simulink model "fixedWingPath"  (R2023b)
settings: Solver=FixedStepAuto  StartTime=0.0  StopTime=70  FixedStep=0.01  RelTol=1e-3
model workspace: external: MATLAB File variable.m (data not in the file)
undefined symbols (not defined in the file or in its folder): DiscIntNeverNeededParam, LOGPOSX, POSY, Tgps, Tneuro, VarImu, VarNeuro
libraries: simulink x2, embmathops x2, uavalgslib x2, robotcorelib x1, uavutilslib x1
(part 1 of 2)
settings Model: DataDictionary=fixedWingPathFollowingData.sldd  EnableAccessToBaseWorkspace=off  PacingRate=10  Creator=The MathWorks, Inc.  LastModifiedBy=Utilisateur
settings SolverCC: AlgebraicLoopSolver=TrustRegion  DecoupledContinuousIntegration=on
settings DataIOCC: ReturnWorkspaceOutputs=off
settings OptimizationCC: ReuseModelBlockBuffer=off
settings DebuggingCC: UnconnectedInputMsg=warning  UnconnectedOutputMsg=warning  UnconnectedLineMsg=warning  ArithmeticOperatorsInVariantConditions=warning
settings ModelReferenceCC: EnableRefExpFcnMdlSchedulingChecks=on
settings SFSimCC: SimUseLocalCustomCode=off  CustomCodeUndefinedFunction=UseInterfaceOnly
settings RTWCC: RTWUseLocalCustomCode=off  DLArmComputeVersion=19.05

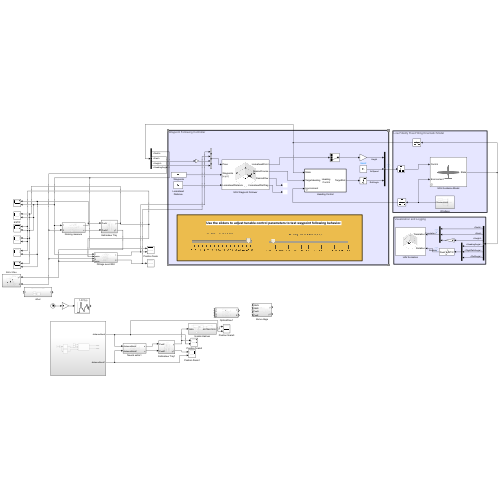
[thumbnail: Simulink's stored preview of the top-level diagram]
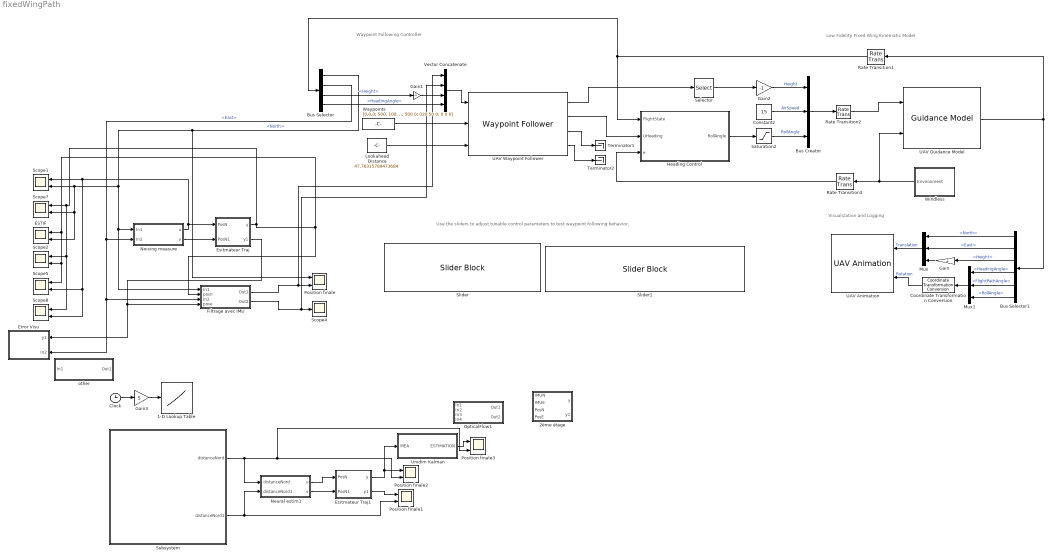
== system fixedWingPath ==
  note: Use the sliders to adjust tunable control parameters to test waypoint following behavior.
  note: Visualization and Logging
  note: Low Fidelity Fixed Wing Kinematic Model
  note: Waypoint Following Controller
  1-D Lookup Table : Lookup_n-D  NumberOfTableDimensions=1  BreakpointsForDimension1=1:337  Table=LOGPOSX  InternalRulePriority=Speed  RndMeth=Simplest
  2ème étage : Subsystem
  Bus Creator : BusCreator  Inputs=3  OutDataTypeStr=Bus: FixedWingControlBus  NonVirtualBus=on
  Bus Selector : BusSelector  OutputSignals=North,East,Height,HeadingAngle
  Bus Selector1 : BusSelector  OutputSignals=North,East,Height,HeadingAngle,FlightPathAngle,RollAngle
  Clock : Clock
  Constant2 : Constant  Value=15
  Coordinate Transformation Conversion : robotcorelib/Coordinate Transformation Conversion  InputRepresentation=Euler Angles  InputEulerSequence=ZYX  ShowTrVecInputPort=on  OutputRepresentation=Quaternion  OutputEulerSequence=ZYX  ShowTrVecOutputPort=on  SimulateUsing=Code generation
  ESTIF : Scope  NumInputPorts=2
  Error Visu : Subsystem
  Esitmateur Traj : Subsystem
  Esitmateur Traj1 : Subsystem
  Filtrage avec IMU : Subsystem
  Gain : Gain  Gain=-1
  Gain1 : Gain  Gain=-1
  Gain2 : Gain  Gain=-1
  Gain3 : Gain  Gain=5
  Heading Control : MATLAB Function  TreatAsAtomicUnit=on  mask(Fixed Wing Heading Controller){PHeadingAngle=0.5997978032950574}
      mask prompts: PHeadingAngle "Heading Control Gain"
      mask help: P controller that regulates fixed wing UAV heading direction through controlling its roll angle. This controller requires that the plane is flying under coordinated flight condition.
  Lookahead Distance : Constant  Value=47.76315789473684
  Mux : Mux  Inputs=3
  Mux1 : Mux  Inputs=3
  Neural estim1 : Subsystem
  Noising measure : Subsystem
  OpticalFlow1 : Subsystem
  Position finale{,1..3} (4 alike) : Scope  NumInputPorts=2
  Rate Transition1 : RateTransition  OutPortSampleTime=0.01
  Rate Transition2 : RateTransition  OutPortSampleTime=0.1
  Rate Transition3 : RateTransition  OutPortSampleTime=0.01
  Saturation2 : Saturate  UpperLimit=20/180*pi  LowerLimit=-20/180*pi
  Scope{1..2,5,7..8} (5 alike) : Scope  NumInputPorts=2
  Scope4 : Scope
  Selector : Selector  InputPortWidth=3  IndexOptions=Index vector (dialog)  Indices=[3]  OutputSizes=1
  Slider : SliderBlock  ScaleMin=5  ScaleMax=50
  Slider1 : SliderBlock  ScaleMin=0.39000000000000001  ScaleMax=3.8999999999999999
  Subsystem : Subsystem
  Terminator1 : Terminator
  Terminator2 : Terminator
  UAV Animation : uavutilslib/UAV Animation  UAVType=FixedWing  UAVSize=50  InertialZDirection=Down  SampleTime=0.1
  UAV Guidance Model : uavalgslib/Guidance Model  ModelType=FixedWingGuidance  SpecifiedDataType=double  SimulateUsing=Code generation  InitialWorldPositionMultirotor=[0; 0; 0]  InitialWorldVelocityMultirotor=[0; 0; 0]  InitialEulerZYXMultirotor=[0; 0; 0]  InitialBodyAngularRateRPYMultirotor=[0; 0; 0]  InitialThrustMultirotor=0  InitialNorthFixedWing=0  InitialEastFixedWing=0  InitialHeightFixedWing=0  InitialAirSpeedFixedWing=15  InitialHeadingAngleFixedWing=0  InitialFlightPathAngleFixedWing=0  InitialRollAngleFixedWing=0  InitialRollAngleRateFixedWing=0  PDRollMultirotor=[3402.97,116.67]  PDPitchMultirotor=[3402.97, 116.67]  PYawRateMultirotor=1950  PThrustMultirotor=3900  MassMultirotor=0.1  PHeightFixedWing=3.9  PHeadingAngleFixedWing=3.9  PFlightPathAngleFixedWing=39  PDRollFixedWing=[5.9414, 3.9]  PAirSpeedFixedWing=1  FlightPathAngleLimitsFixedWing=[-pi/6, pi/6]  StateBusName='FixedWingStateBus'  ControlBusName='FixedWingControlBus'  EnvironmentBusName='FixedWingEnvironmentBus'  DataType=double
  UAV Waypoint Follower : uavalgslib/Waypoint Follower  UAVType=fixed-wing  StartFrom=first  TransitionRadiusSource=internal  TransitionRadius=10  MinLookaheadDistance=0.1  YawInput=off  ShowCrossTrackErrorOutput=off  ShowStatusOutput=off  SimulateUsing=Code generation
  Unidim Kalman : Subsystem
  Vector Concatenate : Concatenate  NumInputs=4
  Waypoints : Constant  Value=[0,0,0; 500, 100, 3; 500, 500, 0; 020 500 0; 020 50 0; 0 0 0]  VectorParams1D=off
  Windless : Subsystem  VariantControl=NoWind
  other : Subsystem
  wires:
  Constant2/1 -> Bus Creator/2  "AirSpeed"
  Gain2/1 -> Bus Creator/1  "Height"
  Bus Creator/1 -> Rate Transition2/1
  Bus Selector/1 -> Position finale/1, ESTIF/2, Scope7/2, Scope1/2, Filtrage avec IMU/1(In1), Noising measure/1(In1)  "<North>"
  Bus Selector/2 -> Error Visu/2(In2), Filtrage avec IMU/3(In2), Noising measure/2(In2)  "<East>"
  Saturation2/1 -> Bus Creator/3  "RollAngle"
  Rate Transition1/1 -> Heading Control/1(FlightState), Bus Selector/1
  Rate Transition2/1 -> UAV Guidance Model/1
  UAV Waypoint Follower/2 -> Heading Control/2(UHeading)
  UAV Waypoint Follower/1 -> Selector/1
  Waypoints/1 -> UAV Waypoint Follower/2
  Vector Concatenate/1 -> UAV Waypoint Follower/1
  UAV Waypoint Follower/3 -> Terminator1/1
  Lookahead Distance/1 -> UAV Waypoint Follower/3
  Heading Control/1(RollAngle) -> Saturation2/1
  Gain/1 -> Mux/3
  Bus Selector1/6 -> Mux1/3  "<RollAngle>"
  Bus Selector1/5 -> Mux1/2  "<FlightPathAngle>"
  Mux1/1 -> Coordinate Transformation Conversion/1
  Coordinate Transformation Conversion/1 -> UAV Animation/2  "Rotation"
  UAV Guidance Model/1 -> Bus Selector1/1, Rate Transition1/1
  Mux/1 -> UAV Animation/1  "Translation"
  Windless/1(Environment) -> UAV Guidance Model/2, Rate Transition3/1
  Bus Selector/4 -> Vector Concatenate/4  "<HeadingAngle>"
  Bus Selector/3 -> Gain1/1  "<Height>"
  Gain1/1 -> Vector Concatenate/3
  Selector/1 -> Gain2/1
  Rate Transition3/1 -> Heading Control/3(e)
  Bus Selector1/1 -> Mux/1  "<North>"
  Bus Selector1/2 -> Mux/2  "<East>"
  Bus Selector1/4 -> Mux1/1  "<HeadingAngle>"
  Bus Selector1/3 -> Gain/1  "<Height>"
  UAV Waypoint Follower/4 -> Terminator2/1
  Filtrage avec IMU/1(Out1) -> Vector Concatenate/1, Position finale/2
  Filtrage avec IMU/2(Out2) -> Vector Concatenate/2, Scope4/1
  Noising measure/1(u) -> Scope8/2, Scope5/2, Scope1/1, Esitmateur Traj/1(PosN)
  Noising measure/2(v) -> Esitmateur Traj/2(PosN1)
  Esitmateur Traj/1(y) -> Scope8/1, Scope2/1, Scope7/1, Scope5/1, Scope2/2, ESTIF/1, Filtrage avec IMU/2(posn)
  Esitmateur Traj/2(y1) -> Filtrage avec IMU/4(pose), Error Visu/1(y1)
  Neural estim1/1(u) -> Esitmateur Traj1/1(PosN)
  Clock/1 -> Gain3/1
  Gain3/1 -> 1-D Lookup Table/1
  Esitmateur Traj1/1(y) -> Unidim Kalman/1(MEA), Position finale2/1
  Esitmateur Traj1/2(y1) -> Position finale1/1
  Neural estim1/2(v) -> Esitmateur Traj1/2(PosN1)
  Subsystem/1(distanceNord) -> Neural estim1/1(distanceNord), Position finale3/2, Position finale2/2
  Subsystem/2(distanceNord1) -> Position finale1/2, Neural estim1/2(distanceNord1)
  Unidim Kalman/1(ESTIMATION) -> Position finale3/1

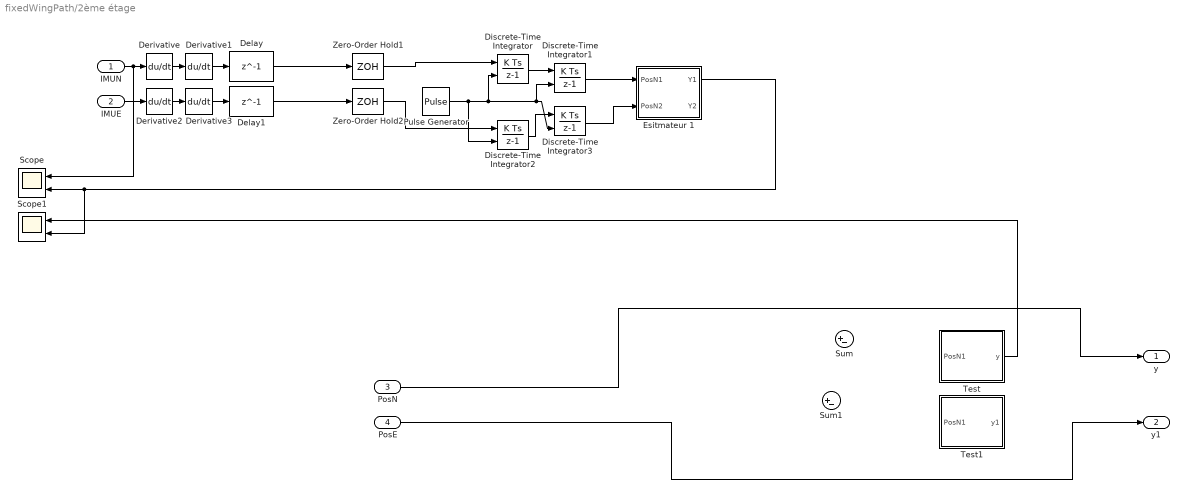
== system fixedWingPath/2ème étage ==
  IMUN : Inport
  IMUE : Inport  Port=2
  PosN : Inport  Port=3
  PosE : Inport  Port=4
  Delay : Delay  DelayLength=1  InitialCondition=0  SampleTime=0.05
  Delay1 : Delay  DelayLength=1  InitialCondition=0  SampleTime=0.05
  Derivative{,1..3} (4 alike) : Derivative
  Discrete-Time Integrator{,1..3} (4 alike) : DiscreteIntegrator  ExternalReset=rising  SampleTime=0.1  ICPrevOutput=DiscIntNeverNeededParam  ICPrevScaledInput=DiscIntNeverNeededParam
  Esitmateur 1 : Subsystem
  Pulse Generator : DiscretePulseGenerator  PulseType=Time based  Period=Tneuro  PulseWidth=50
  Scope : Scope  NumInputPorts=2
  Scope1 : Scope  NumInputPorts=2
  Sum : Sum  Inputs=|+-
  Sum1 : Sum  Inputs=|+-
  Test : Subsystem
  Test1 : Subsystem
  Zero-Order Hold1 : ZeroOrderHold  SampleTime=Tgps
  Zero-Order Hold2 : ZeroOrderHold  SampleTime=Tgps
  y : Outport
  y1 : Outport  Port=2
  wires:
  Zero-Order Hold1/1 -> Discrete-Time Integrator/1
  Derivative1/1 -> Delay/1
  Derivative/1 -> Derivative1/1
  IMUN/1 -> Scope/1, Derivative/1
  Derivative3/1 -> Delay1/1
  Zero-Order Hold2/1 -> Discrete-Time Integrator2/1
  IMUE/1 -> Derivative2/1
  Derivative2/1 -> Derivative3/1
  Pulse Generator/1 -> Discrete-Time Integrator2/2, Discrete-Time Integrator3/2, Discrete-Time Integrator1/2, Discrete-Time Integrator/2
  Discrete-Time Integrator/1 -> Discrete-Time Integrator1/1
  Discrete-Time Integrator2/1 -> Discrete-Time Integrator3/1
  Discrete-Time Integrator1/1 -> Esitmateur 1/1(PosN1)
  Discrete-Time Integrator3/1 -> Esitmateur 1/2(PosN2)
  Esitmateur 1/1(Y1) -> Scope1/2, Scope/2
  Delay/1 -> Zero-Order Hold1/1
  Delay1/1 -> Zero-Order Hold2/1
  Test/1(y) -> Scope1/1
  PosN/1 -> y/1
  PosE/1 -> y1/1

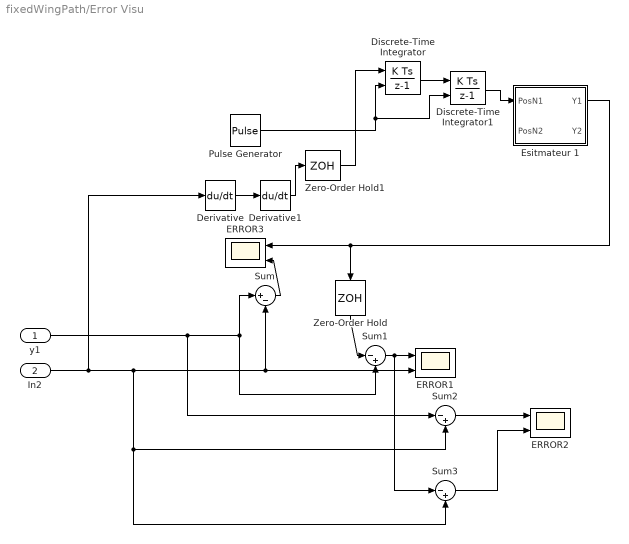
== system fixedWingPath/Error Visu ==
  y1 : Inport
  In2 : Inport  Port=2
  Derivative : Derivative
  Derivative1 : Derivative
  Discrete-Time Integrator : DiscreteIntegrator  ExternalReset=rising  SampleTime=0.1  ICPrevOutput=DiscIntNeverNeededParam  ICPrevScaledInput=DiscIntNeverNeededParam
  Discrete-Time Integrator1 : DiscreteIntegrator  ExternalReset=rising  SampleTime=0.1  ICPrevOutput=DiscIntNeverNeededParam  ICPrevScaledInput=DiscIntNeverNeededParam
  ERROR1 : Scope  NumInputPorts=2
  ERROR2 : Scope  NumInputPorts=2
  ERROR3 : Scope  NumInputPorts=2
  Esitmateur 1 : Subsystem
  Pulse Generator : DiscretePulseGenerator  PulseType=Time based  Period=Tneuro  PulseWidth=50
  Sum : Sum  Inputs=|+-
  Sum1 : Sum  Inputs=|-+
  Sum2 : Sum  Inputs=|-+
  Sum3 : Sum  Inputs=|-+
  Zero-Order Hold : ZeroOrderHold  SampleTime=Tgps
  Zero-Order Hold1 : ZeroOrderHold  SampleTime=Tgps
  wires:
  Sum/1 -> ERROR3/2
  y1/1 -> Sum/1, Sum1/2, Sum2/1
  In2/1 -> Sum2/2, Sum3/2, ERROR1/2, Sum/2, Derivative/1
  Derivative1/1 -> Zero-Order Hold1/1
  Sum1/1 -> Sum3/1, ERROR1/1
  Zero-Order Hold/1 -> Sum1/1
  Derivative/1 -> Derivative1/1
  Zero-Order Hold1/1 -> Discrete-Time Integrator/1
  Sum2/1 -> ERROR2/1
  Sum3/1 -> ERROR2/2
  Discrete-Time Integrator/1 -> Discrete-Time Integrator1/1
  Pulse Generator/1 -> Discrete-Time Integrator/2, Discrete-Time Integrator1/2
  Discrete-Time Integrator1/1 -> Esitmateur 1/1(PosN1)
  Esitmateur 1/1(Y1) -> Zero-Order Hold/1, ERROR3/1

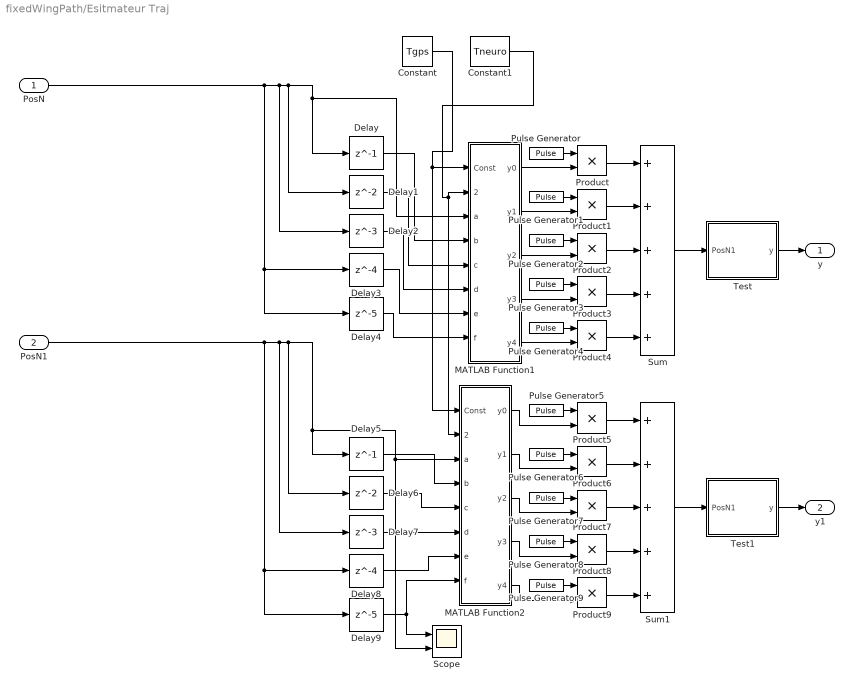
== system fixedWingPath/Esitmateur Traj ==
  PosN : Inport
  PosN1 : Inport  Port=2
  Constant : Constant  Value=Tgps
  Constant1 : Constant  Value=Tneuro
  Delay : Delay  DelayLength=1  SampleTime=Tneuro
  Delay1 : Delay  SampleTime=Tneuro
  Delay2 : Delay  DelayLength=3  SampleTime=Tneuro
  Delay3 : Delay  DelayLength=4  SampleTime=Tneuro
  Delay4 : Delay  DelayLength=5  SampleTime=Tneuro
  Delay5 : Delay  DelayLength=1  SampleTime=Tneuro
  Delay6 : Delay  SampleTime=Tneuro
  Delay7 : Delay  DelayLength=3  SampleTime=Tneuro
  Delay8 : Delay  DelayLength=4  SampleTime=Tneuro
  Delay9 : Delay  DelayLength=5  SampleTime=Tneuro
  MATLAB Function1 : MATLAB Function  TreatAsAtomicUnit=on
  MATLAB Function2 : MATLAB Function  TreatAsAtomicUnit=on
  Product{,1..9} (10 alike) : Product
  Pulse Generator : DiscretePulseGenerator  PulseType=Time based  Period=Tneuro  PulseWidth=20
  Pulse Generator1 : DiscretePulseGenerator  PulseType=Time based  Period=Tneuro  PulseWidth=20  PhaseDelay=0.2*Tneuro
  Pulse Generator2 : DiscretePulseGenerator  PulseType=Time based  Period=Tneuro  PulseWidth=20  PhaseDelay=0.4*Tneuro
  Pulse Generator3 : DiscretePulseGenerator  PulseType=Time based  Period=Tneuro  PulseWidth=20  PhaseDelay=0.6*Tneuro
  Pulse Generator4 : DiscretePulseGenerator  PulseType=Time based  Period=Tneuro  PulseWidth=20  PhaseDelay=0.8*Tneuro
  Pulse Generator5 : DiscretePulseGenerator  PulseType=Time based  Period=Tneuro  PulseWidth=20
  Pulse Generator6 : DiscretePulseGenerator  PulseType=Time based  Period=Tneuro  PulseWidth=20  PhaseDelay=0.2*Tneuro
  Pulse Generator7 : DiscretePulseGenerator  PulseType=Time based  Period=Tneuro  PulseWidth=20  PhaseDelay=0.4*Tneuro
  Pulse Generator8 : DiscretePulseGenerator  PulseType=Time based  Period=Tneuro  PulseWidth=20  PhaseDelay=0.6*Tneuro
  Pulse Generator9 : DiscretePulseGenerator  PulseType=Time based  Period=Tneuro  PulseWidth=20  PhaseDelay=0.8*Tneuro
  Scope : Scope  NumInputPorts=2
  Sum : Sum  Inputs=+++++
  Sum1 : Sum  Inputs=+++++
  Test : Subsystem
  Test1 : Subsystem
  y : Outport
  y1 : Outport  Port=2
  wires:
  Delay/1 -> MATLAB Function1/4(b)
  Delay1/1 -> MATLAB Function1/5(c)
  Delay2/1 -> MATLAB Function1/6(d)
  Delay3/1 -> MATLAB Function1/7(e)
  Delay4/1 -> MATLAB Function1/8(f)
  Product/1 -> Sum/1
  Product1/1 -> Sum/2
  Product2/1 -> Sum/3
  Product3/1 -> Sum/4
  Product4/1 -> Sum/5
  Pulse Generator/1 -> Product/1
  Pulse Generator1/1 -> Product1/1
  Pulse Generator2/1 -> Product2/1
  Pulse Generator3/1 -> Product3/1
  Pulse Generator4/1 -> Product4/1
  MATLAB Function1/1(y0) -> Product/2
  MATLAB Function1/2(y1) -> Product1/2
  MATLAB Function1/3(y2) -> Product2/2
  MATLAB Function1/4(y3) -> Product3/2
  MATLAB Function1/5(y4) -> Product4/2
  MATLAB Function2/3(y2) -> Product7/2
  Product9/1 -> Sum1/5
  Product7/1 -> Sum1/3
  MATLAB Function2/2(y1) -> Product6/2
  Product8/1 -> Sum1/4
  MATLAB Function2/5(y4) -> Product9/2
  Pulse Generator6/1 -> Product6/1
  Product6/1 -> Sum1/2
  Pulse Generator9/1 -> Product9/1
  Pulse Generator7/1 -> Product7/1
  Pulse Generator8/1 -> Product8/1
  Product5/1 -> Sum1/1
  MATLAB Function2/4(y3) -> Product8/2
  Pulse Generator5/1 -> Product5/1
  MATLAB Function2/1(y0) -> Product5/2
  Constant/1 -> MATLAB Function2/1(Const), MATLAB Function1/1(Const)
  Delay5/1 -> MATLAB Function2/4(b)
  Delay6/1 -> MATLAB Function2/5(c)
  Delay7/1 -> MATLAB Function2/6(d)
  Delay8/1 -> MATLAB Function2/7(e)
  Delay9/1 -> MATLAB Function2/8(f), Scope/1
  Constant1/1 -> MATLAB Function2/2(Const2), MATLAB Function1/2(Const2)
  PosN1/1 -> Delay9/1, Delay8/1, Delay7/1, Delay6/1, MATLAB Function2/3(a), Scope/2, Delay5/1
  PosN/1 -> Delay4/1, Delay3/1, Delay2/1, Delay1/1, Delay/1, MATLAB Function1/3(a)
  Sum/1 -> Test/1(PosN1)
  Test/1(y) -> y/1
  Test1/1(y) -> y1/1
  Sum1/1 -> Test1/1(PosN1)

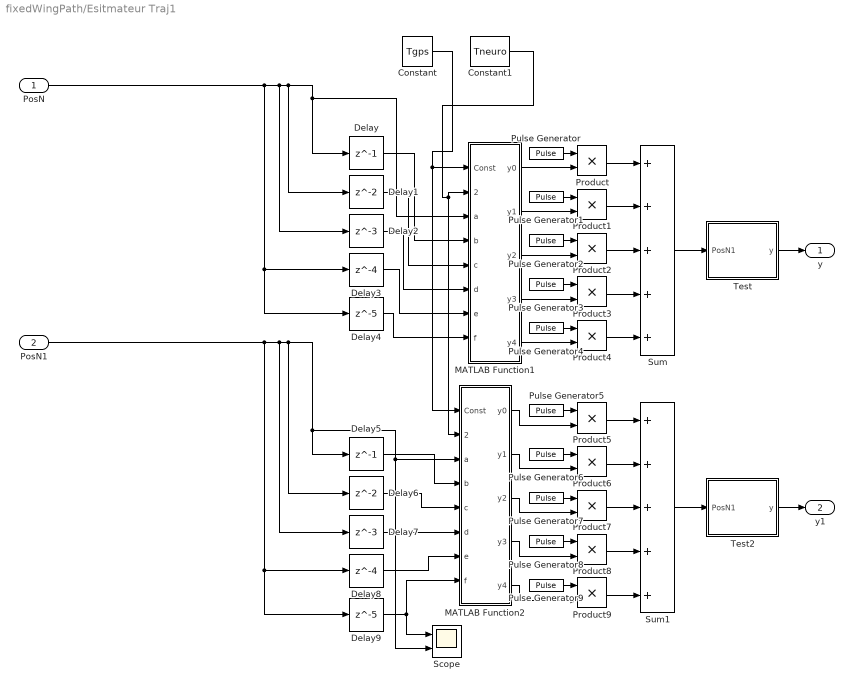
== system fixedWingPath/Esitmateur Traj1 ==
  PosN : Inport
  PosN1 : Inport  Port=2
  Constant : Constant  Value=Tgps
  Constant1 : Constant  Value=Tneuro
  Delay : Delay  DelayLength=1  SampleTime=Tneuro
  Delay1 : Delay  SampleTime=Tneuro
  Delay2 : Delay  DelayLength=3  SampleTime=Tneuro
  Delay3 : Delay  DelayLength=4  SampleTime=Tneuro
  Delay4 : Delay  DelayLength=5  SampleTime=Tneuro
  Delay5 : Delay  DelayLength=1  SampleTime=Tneuro
  Delay6 : Delay  SampleTime=Tneuro
  Delay7 : Delay  DelayLength=3  SampleTime=Tneuro
  Delay8 : Delay  DelayLength=4  SampleTime=Tneuro
  Delay9 : Delay  DelayLength=5  SampleTime=Tneuro
  MATLAB Function1 : MATLAB Function  TreatAsAtomicUnit=on
  MATLAB Function2 : MATLAB Function  TreatAsAtomicUnit=on
  Product{,1..9} (10 alike) : Product
  Pulse Generator : DiscretePulseGenerator  PulseType=Time based  Period=Tneuro  PulseWidth=20
  Pulse Generator1 : DiscretePulseGenerator  PulseType=Time based  Period=Tneuro  PulseWidth=20  PhaseDelay=0.2*Tneuro
  Pulse Generator2 : DiscretePulseGenerator  PulseType=Time based  Period=Tneuro  PulseWidth=20  PhaseDelay=0.4*Tneuro
  Pulse Generator3 : DiscretePulseGenerator  PulseType=Time based  Period=Tneuro  PulseWidth=20  PhaseDelay=0.6*Tneuro
  Pulse Generator4 : DiscretePulseGenerator  PulseType=Time based  Period=Tneuro  PulseWidth=20  PhaseDelay=0.8*Tneuro
  Pulse Generator5 : DiscretePulseGenerator  PulseType=Time based  Period=Tneuro  PulseWidth=20
  Pulse Generator6 : DiscretePulseGenerator  PulseType=Time based  Period=Tneuro  PulseWidth=20  PhaseDelay=0.2*Tneuro
  Pulse Generator7 : DiscretePulseGenerator  PulseType=Time based  Period=Tneuro  PulseWidth=20  PhaseDelay=0.4*Tneuro
  Pulse Generator8 : DiscretePulseGenerator  PulseType=Time based  Period=Tneuro  PulseWidth=20  PhaseDelay=0.6*Tneuro
  Pulse Generator9 : DiscretePulseGenerator  PulseType=Time based  Period=Tneuro  PulseWidth=20  PhaseDelay=0.8*Tneuro
  Scope : Scope  NumInputPorts=2
  Sum : Sum  Inputs=+++++
  Sum1 : Sum  Inputs=+++++
  Test : Subsystem
  Test2 : Subsystem
  y : Outport
  y1 : Outport  Port=2
  wires:
  Delay/1 -> MATLAB Function1/4(b)
  Delay1/1 -> MATLAB Function1/5(c)
  Delay2/1 -> MATLAB Function1/6(d)
  Delay3/1 -> MATLAB Function1/7(e)
  Delay4/1 -> MATLAB Function1/8(f)
  Product/1 -> Sum/1
  Product1/1 -> Sum/2
  Product2/1 -> Sum/3
  Product3/1 -> Sum/4
  Product4/1 -> Sum/5
  Pulse Generator/1 -> Product/1
  Pulse Generator1/1 -> Product1/1
  Pulse Generator2/1 -> Product2/1
  Pulse Generator3/1 -> Product3/1
  Pulse Generator4/1 -> Product4/1
  MATLAB Function1/1(y0) -> Product/2
  MATLAB Function1/2(y1) -> Product1/2
  MATLAB Function1/3(y2) -> Product2/2
  MATLAB Function1/4(y3) -> Product3/2
  MATLAB Function1/5(y4) -> Product4/2
  MATLAB Function2/3(y2) -> Product7/2
  Product9/1 -> Sum1/5
  Product7/1 -> Sum1/3
  MATLAB Function2/2(y1) -> Product6/2
  Product8/1 -> Sum1/4
  MATLAB Function2/5(y4) -> Product9/2
  Pulse Generator6/1 -> Product6/1
  Product6/1 -> Sum1/2
  Pulse Generator9/1 -> Product9/1
  Pulse Generator7/1 -> Product7/1
  Pulse Generator8/1 -> Product8/1
  Product5/1 -> Sum1/1
  MATLAB Function2/4(y3) -> Product8/2
  Pulse Generator5/1 -> Product5/1
  MATLAB Function2/1(y0) -> Product5/2
  Constant/1 -> MATLAB Function2/1(Const), MATLAB Function1/1(Const)
  Delay5/1 -> MATLAB Function2/4(b)
  Delay6/1 -> MATLAB Function2/5(c)
  Delay7/1 -> MATLAB Function2/6(d)
  Delay8/1 -> MATLAB Function2/7(e)
  Delay9/1 -> MATLAB Function2/8(f), Scope/1
  Constant1/1 -> MATLAB Function2/2(Const2), MATLAB Function1/2(Const2)
  PosN1/1 -> Delay9/1, Delay8/1, Delay7/1, Delay6/1, MATLAB Function2/3(a), Scope/2, Delay5/1
  PosN/1 -> Delay4/1, Delay3/1, Delay2/1, Delay1/1, Delay/1, MATLAB Function1/3(a)
  Sum/1 -> Test/1(PosN1)
  Test/1(y) -> y/1
  Test2/1(y) -> y1/1
  Sum1/1 -> Test2/1(PosN1)

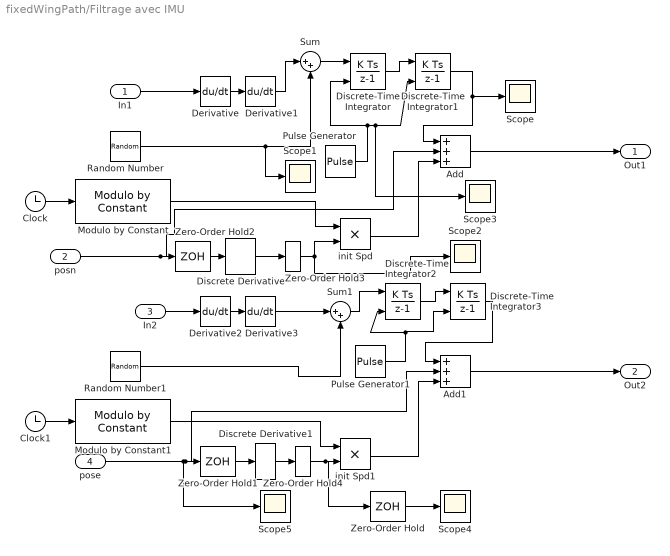
== system fixedWingPath/Filtrage avec IMU ==
  In1 : Inport
  posn : Inport  Port=2
  In2 : Inport  Port=3
  pose : Inport  Port=4
  Add : Sum  Inputs=+++
  Add1 : Sum  Inputs=+++
  Clock : Clock
  Clock1 : Clock
  Derivative{,1..3} (4 alike) : Derivative
  Discrete Derivative : simulink/Discrete/Discrete Derivative  gainval=1.0  ICPrevScaledInput=0.0  OutMin=[]  OutMax=[]  OutDataType=fixdt(1, 16)  OutScaling=2^-10  DoSatur=off
  Discrete Derivative1 : simulink/Discrete/Discrete Derivative  gainval=1.0  ICPrevScaledInput=0.0  OutMin=[]  OutMax=[]  OutDataType=fixdt(1, 16)  OutScaling=2^-10  DoSatur=off
  Discrete-Time Integrator{,1..3} (4 alike) : DiscreteIntegrator  ExternalReset=rising  SampleTime=0.01  ICPrevOutput=DiscIntNeverNeededParam  ICPrevScaledInput=DiscIntNeverNeededParam
  Modulo by Constant : embmathops/Modulo by Constant  Denominator=Tgps  SimulateUsing=Code generation
      settings: LibrarySourceBlock=embeddedMathLib/Modulo by Constant
  Modulo by Constant1 : embmathops/Modulo by Constant  Denominator=Tgps  SimulateUsing=Code generation
      settings: LibrarySourceBlock=embeddedMathLib/Modulo by Constant
  Pulse Generator : DiscretePulseGenerator  PulseType=Time based  Period=Tgps  PulseWidth=50
  Pulse Generator1 : DiscretePulseGenerator  PulseType=Time based  Period=Tgps  PulseWidth=50
  Random Number : RandomNumber  Variance=1*VarImu  SampleTime=0.1
  Random Number1 : RandomNumber  Variance=1*VarImu  SampleTime=0.1
  Scope{,1..5} (6 alike) : Scope
  Sum : Sum  Inputs=|++
  Sum1 : Sum  Inputs=|++
  Zero-Order Hold : ZeroOrderHold  SampleTime=Tgps
  Zero-Order Hold1 : ZeroOrderHold  SampleTime=Tneuro
  Zero-Order Hold2 : ZeroOrderHold  SampleTime=Tneuro
  Zero-Order Hold3 : ZeroOrderHold  SampleTime=Tgps
  Zero-Order Hold4 : ZeroOrderHold  SampleTime=Tgps
  init Spd : Product
  init Spd1 : Product
  Out1 : Outport
  Out2 : Outport  Port=2
  wires:
  Derivative/1 -> Derivative1/1
  In1/1 -> Derivative/1
  Add/1 -> Out1/1
  Derivative1/1 -> Sum/1
  Clock/1 -> Modulo by Constant/1
  Modulo by Constant/1 -> init Spd/1
  Random Number/1 -> Scope1/1, Sum/2
  Discrete Derivative/1 -> Zero-Order Hold3/1
  init Spd/1 -> Add/3
  posn/1 -> Add/2, Zero-Order Hold2/1
  Sum/1 -> Discrete-Time Integrator/1
  Discrete-Time Integrator/1 -> Discrete-Time Integrator1/1
  Discrete-Time Integrator1/1 -> Add/1, Scope/1
  Sum1/1 -> Discrete-Time Integrator2/1
  Derivative3/1 -> Sum1/1
  Modulo by Constant1/1 -> init Spd1/1
  init Spd1/1 -> Add1/3
  pose/1 -> Zero-Order Hold1/1, Add1/2, Scope5/1
  Discrete Derivative1/1 -> Zero-Order Hold4/1
  Add1/1 -> Out2/1
  Clock1/1 -> Modulo by Constant1/1
  Derivative2/1 -> Derivative3/1
  Random Number1/1 -> Sum1/2
  In2/1 -> Derivative2/1
  Discrete-Time Integrator2/1 -> Discrete-Time Integrator3/1
  Discrete-Time Integrator3/1 -> Add1/1
  Pulse Generator/1 -> Scope3/1, Discrete-Time Integrator1/2, Discrete-Time Integrator/2
  Pulse Generator1/1 -> Discrete-Time Integrator3/2, Discrete-Time Integrator2/2
  Zero-Order Hold/1 -> Scope4/1
  Zero-Order Hold1/1 -> Discrete Derivative1/1
  Zero-Order Hold2/1 -> Discrete Derivative/1
  Zero-Order Hold3/1 -> Scope2/1, init Spd/2
  Zero-Order Hold4/1 -> Zero-Order Hold/1, init Spd1/2

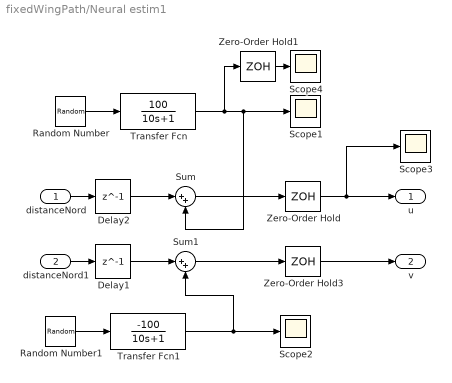
== system fixedWingPath/Neural estim1 ==
  distanceNord : Inport
  distanceNord1 : Inport  Port=2
  Delay1 : Delay  DelayLength=1
  Delay2 : Delay  DelayLength=1
  Random Number : RandomNumber  Variance=1*VarNeuro  SampleTime=0.1
  Random Number1 : RandomNumber  Variance=1*VarNeuro  SampleTime=0.1
  Scope{1..4} (4 alike) : Scope
  Sum : Sum  Inputs=|++
  Sum1 : Sum  Inputs=|++
  Transfer Fcn : TransferFcn  Numerator=[100]  Denominator=[10 1]
  Transfer Fcn1 : TransferFcn  Numerator=[-100]  Denominator=[10 1]
  Zero-Order Hold : ZeroOrderHold  SampleTime=Tneuro
  Zero-Order Hold1 : ZeroOrderHold  SampleTime=Tneuro
  Zero-Order Hold3 : ZeroOrderHold  SampleTime=Tneuro
  u : Outport
  v : Outport  Port=2
  wires:
  distanceNord/1 -> Delay2/1
  Zero-Order Hold/1 -> Scope3/1, u/1
  Zero-Order Hold3/1 -> v/1
  Random Number/1 -> Transfer Fcn/1
  Transfer Fcn/1 -> Zero-Order Hold1/1, Sum/2, Scope1/1
  Sum/1 -> Zero-Order Hold/1
  distanceNord1/1 -> Delay1/1
  Sum1/1 -> Zero-Order Hold3/1
  Transfer Fcn1/1 -> Sum1/2, Scope2/1
  Random Number1/1 -> Transfer Fcn1/1
  Delay2/1 -> Sum/1
  Delay1/1 -> Sum1/1
  Zero-Order Hold1/1 -> Scope4/1

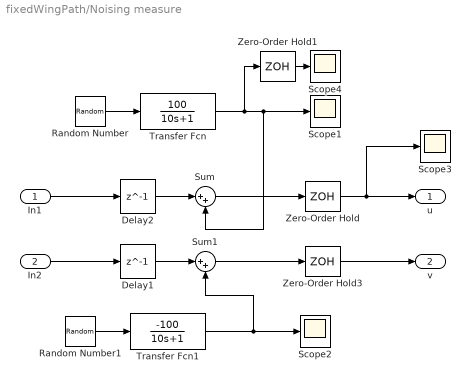
== system fixedWingPath/Noising measure ==
  In1 : Inport
  In2 : Inport  Port=2
  Delay1 : Delay  DelayLength=1  SampleTime=Tneuro
  Delay2 : Delay  DelayLength=1  SampleTime=Tneuro
  Random Number : RandomNumber  Variance=1*VarNeuro  SampleTime=0.1
  Random Number1 : RandomNumber  Variance=1*VarNeuro  SampleTime=0.1
  Scope{1..4} (4 alike) : Scope
  Sum : Sum  Inputs=|++
  Sum1 : Sum  Inputs=|++
  Transfer Fcn : TransferFcn  Numerator=[100]  Denominator=[10 1]
  Transfer Fcn1 : TransferFcn  Numerator=[-100]  Denominator=[10 1]
  Zero-Order Hold : ZeroOrderHold  SampleTime=Tneuro
  Zero-Order Hold1 : ZeroOrderHold  SampleTime=Tneuro
  Zero-Order Hold3 : ZeroOrderHold  SampleTime=Tneuro
  u : Outport
  v : Outport  Port=2
  wires:
  Zero-Order Hold/1 -> Scope3/1, u/1
  Zero-Order Hold3/1 -> v/1
  Random Number/1 -> Transfer Fcn/1
  Transfer Fcn/1 -> Zero-Order Hold1/1, Sum/2, Scope1/1
  Sum/1 -> Zero-Order Hold/1
  Sum1/1 -> Zero-Order Hold3/1
  Transfer Fcn1/1 -> Sum1/2, Scope2/1
  Random Number1/1 -> Transfer Fcn1/1
  Delay2/1 -> Sum/1
  Delay1/1 -> Sum1/1
  Zero-Order Hold1/1 -> Scope4/1
  In1/1 -> Delay2/1
  In2/1 -> Delay1/1

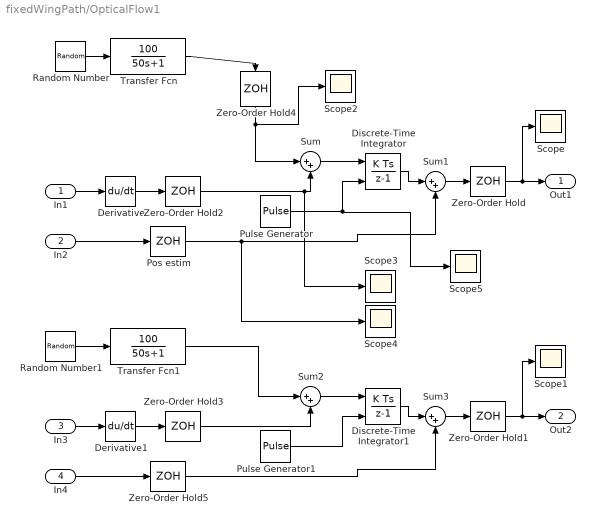
== system fixedWingPath/OpticalFlow1 ==
  In1 : Inport
  In2 : Inport  Port=2
  In3 : Inport  Port=3
  In4 : Inport  Port=4
  Derivative : Derivative
  Derivative1 : Derivative
  Discrete-Time Integrator : DiscreteIntegrator  ExternalReset=rising  SampleTime=0.01  ICPrevOutput=DiscIntNeverNeededParam  ICPrevScaledInput=DiscIntNeverNeededParam
  Discrete-Time Integrator1 : DiscreteIntegrator  ExternalReset=rising  SampleTime=0.01  ICPrevOutput=DiscIntNeverNeededParam  ICPrevScaledInput=DiscIntNeverNeededParam
  Pos estim : ZeroOrderHold
  Pulse Generator : DiscretePulseGenerator  PulseType=Time based  Period=1  PulseWidth=50
  Pulse Generator1 : DiscretePulseGenerator  PulseType=Time based  Period=1  PulseWidth=50
  Random Number : RandomNumber  SampleTime=0.1
  Random Number1 : RandomNumber  SampleTime=0.1
  Scope{,1..5} (6 alike) : Scope
  Sum{,1..3} (4 alike) : Sum  Inputs=|++
  Transfer Fcn : TransferFcn  Numerator=[100]  Denominator=[50 1]
  Transfer Fcn1 : TransferFcn  Numerator=[100]  Denominator=[50 1]
  Zero-Order Hold{,1..4} (5 alike) : ZeroOrderHold  SampleTime=0.1
  Zero-Order Hold5 : ZeroOrderHold
  Out1 : Outport
  Out2 : Outport  Port=2
  wires:
  Sum1/1 -> Zero-Order Hold/1
  Random Number/1 -> Transfer Fcn/1
  Transfer Fcn/1 -> Zero-Order Hold4/1
  In1/1 -> Derivative/1
  Derivative/1 -> Zero-Order Hold2/1
  Zero-Order Hold2/1 -> Scope3/1, Sum/2
  Sum/1 -> Discrete-Time Integrator/1
  Pulse Generator/1 -> Discrete-Time Integrator/2, Scope5/1
  Discrete-Time Integrator/1 -> Sum1/1
  In2/1 -> Pos estim/1
  Zero-Order Hold/1 -> Scope/1, Out1/1
  Zero-Order Hold1/1 -> Scope1/1, Out2/1
  Derivative1/1 -> Zero-Order Hold3/1
  Zero-Order Hold3/1 -> Sum2/2
  Sum2/1 -> Discrete-Time Integrator1/1
  Sum3/1 -> Zero-Order Hold1/1
  Transfer Fcn1/1 -> Sum2/1
  In3/1 -> Derivative1/1
  In4/1 -> Zero-Order Hold5/1
  Discrete-Time Integrator1/1 -> Sum3/1
  Pulse Generator1/1 -> Discrete-Time Integrator1/2
  Random Number1/1 -> Transfer Fcn1/1
  Pos estim/1 -> Scope4/1, Sum1/2
  Zero-Order Hold5/1 -> Sum3/2
  Zero-Order Hold4/1 -> Scope2/1, Sum/1

== system fixedWingPath/Subsystem ==
  1-D Lookup Table : Lookup_n-D  NumberOfTableDimensions=1  BreakpointsForDimension1=1:337  Table=LOGPOSX  InternalRulePriority=Speed  RndMeth=Simplest
  1-D Lookup Table1 : Lookup_n-D  NumberOfTableDimensions=1  BreakpointsForDimension1=1:337  Table=POSY  InternalRulePriority=Speed  RndMeth=Simplest
  Clock : Clock
  Constant : Constant  Value=43.4964106
  Constant1 : Constant  Value=1.4991177
  Gain3 : Gain  Gain=5
  MATLAB Function : MATLAB Function  TreatAsAtomicUnit=on
  distanceNord : Outport
  distanceNord1 : Outport  Port=2
  wires:
  Constant1/1 -> MATLAB Function/2(lon1)
  Constant/1 -> MATLAB Function/1(lat1)
  Clock/1 -> Gain3/1
  Gain3/1 -> 1-D Lookup Table1/1, 1-D Lookup Table/1
  1-D Lookup Table/1 -> MATLAB Function/3(lat2)
  1-D Lookup Table1/1 -> MATLAB Function/4(lon2)
  MATLAB Function/1(distanceNord) -> distanceNord/1
  MATLAB Function/2(distanceEst) -> distanceNord1/1

== system fixedWingPath/Unidim Kalman ==
  MEA : Inport
  Constant : Constant
  Delay : Delay  DelayLength=1  InitialCondition=0  SampleTime=Tgps
  Delay1 : Delay  DelayLength=1  InitialCondition=0  SampleTime=Tgps
  MATLAB Function : MATLAB Function  TreatAsAtomicUnit=on
  Step : Step  Before=1  After=0  SampleTime=0.2
  ESTIMATION : Outport
  wires:
  MEA/1 -> MATLAB Function/1(MEA)
  Delay/1 -> MATLAB Function/2(Et1n)
  MATLAB Function/2(Et1) -> Delay/1
  MATLAB Function/1(Estimation) -> ESTIMATION/1, Delay1/1
  Delay1/1 -> MATLAB Function/4(Est1n)
  Constant/1 -> MATLAB Function/3(Emea)
  Step/1 -> MATLAB Function/5(trig)

== system fixedWingPath/Windless ==
  Bus Creator : BusCreator  Inputs=4  OutDataTypeStr=Bus: FixedWingEnvironmentBus  NonVirtualBus=on
  Constant : Constant  Value=9.8066
  Constant3 : Constant  Value=0
  WIND GENERATOR : Subsystem
  WIND GENERATOR1 : Subsystem
  Environment : Outport  VectorParamsAs1DForOutWhenUnconnected=off
  wires:
  WIND GENERATOR1/1(Out1) -> Bus Creator/2  "WindEast"
  Constant3/1 -> Bus Creator/3  "WindDown"
  WIND GENERATOR/1(Out1) -> Bus Creator/1  "WindNorth"
  Bus Creator/1 -> Environment/1
  Constant/1 -> Bus Creator/4  "Gravity"

== system fixedWingPath/other ==
  In1 : Inport
  Discrete Filter : DiscreteFilter  Numerator=[10]  Denominator=[10 0.005 0.001]
  Discrete Filter1 : DiscreteFilter  Numerator=[10]  Denominator=[10 0.005 0.001]
  Filtrage IMU : Subsystem
  Out1 : Outport
  wires:
  In1/1 -> Out1/1
  Discrete Filter1/1 -> Filtrage IMU/2(PosN2)
  Discrete Filter/1 -> Filtrage IMU/1(PosN1)

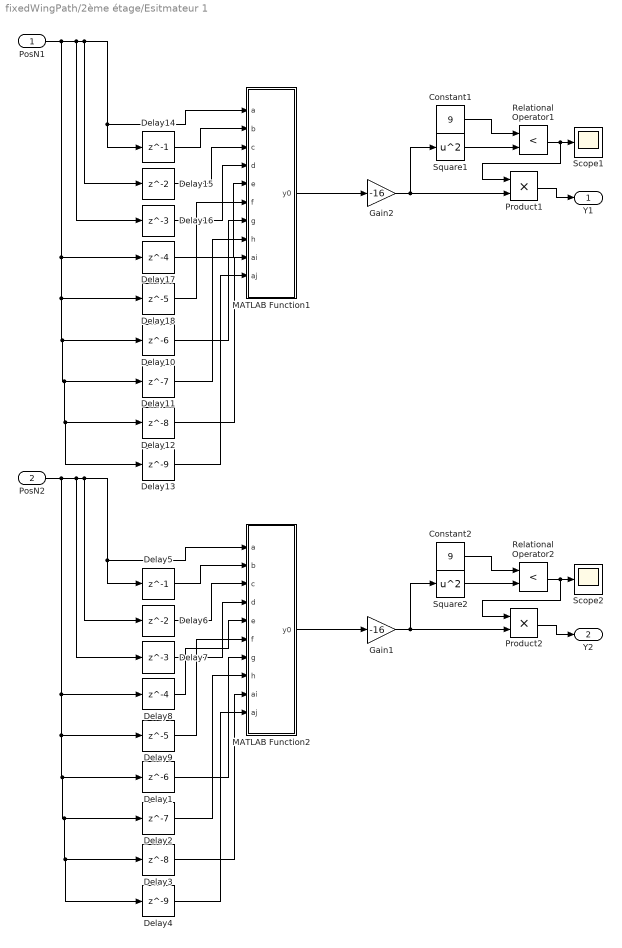
== system fixedWingPath/2ème étage/Esitmateur 1 ==
  PosN1 : Inport
  PosN2 : Inport  Port=2
  Constant1 : Constant  Value=9
  Constant2 : Constant  Value=9
  Delay1 : Delay  DelayLength=6  SampleTime=Tgps
  Delay10 : Delay  DelayLength=6  SampleTime=Tgps
  Delay11 : Delay  DelayLength=7  SampleTime=Tgps
  Delay12 : Delay  DelayLength=8  SampleTime=Tgps
  Delay13 : Delay  DelayLength=9  SampleTime=Tgps
  Delay14 : Delay  DelayLength=1  SampleTime=Tgps
  Delay15 : Delay  SampleTime=Tgps
  Delay16 : Delay  DelayLength=3  SampleTime=Tgps
  Delay17 : Delay  DelayLength=4  SampleTime=Tgps
  Delay18 : Delay  DelayLength=5  SampleTime=Tgps
  Delay2 : Delay  DelayLength=7  SampleTime=Tgps
  Delay3 : Delay  DelayLength=8  SampleTime=Tgps
  Delay4 : Delay  DelayLength=9  SampleTime=Tgps
  Delay5 : Delay  DelayLength=1  SampleTime=Tgps
  Delay6 : Delay  SampleTime=Tgps
  Delay7 : Delay  DelayLength=3  SampleTime=Tgps
  Delay8 : Delay  DelayLength=4  SampleTime=Tgps
  Delay9 : Delay  DelayLength=5  SampleTime=Tgps
  Gain1 : Gain  Gain=-16
  Gain2 : Gain  Gain=-16
  MATLAB Function1 : MATLAB Function  TreatAsAtomicUnit=on
  MATLAB Function2 : MATLAB Function  TreatAsAtomicUnit=on
  Product1 : Product
  Product2 : Product
  Relational Operator1 : RelationalOperator  Operator=<  OutDataTypeStr=boolean  RndMeth=Simplest  InputSameDT=off
  Relational Operator2 : RelationalOperator  Operator=<  OutDataTypeStr=boolean  RndMeth=Simplest  InputSameDT=off
  Scope1 : Scope
  Scope2 : Scope
  Square1 : Math  Operator=square
  Square2 : Math  Operator=square
  Y1 : Outport
  Y2 : Outport  Port=2
  wires:
  Relational Operator1/1 -> Product1/1, Scope1/1
  Constant1/1 -> Relational Operator1/1
  Delay12/1 -> MATLAB Function1/9(ai)
  Delay13/1 -> MATLAB Function1/10(aj)
  Square1/1 -> Relational Operator1/2
  Delay14/1 -> MATLAB Function1/2(b)
  Delay10/1 -> MATLAB Function1/7(g)
  Delay17/1 -> MATLAB Function1/5(e)
  PosN1/1 -> Delay13/1, Delay12/1, Delay11/1, Delay10/1, Delay18/1, Delay17/1, Delay16/1, Delay15/1, MATLAB Function1/1(a), Delay14/1
  Delay11/1 -> MATLAB Function1/8(h)
  Gain2/1 -> Product1/2, Square1/1
  MATLAB Function1/1(y0) -> Gain2/1
  Delay15/1 -> MATLAB Function1/3(c)
  Delay18/1 -> MATLAB Function1/6(f)
  Delay16/1 -> MATLAB Function1/4(d)
  Product1/1 -> Y1/1
  PosN2/1 -> Delay4/1, Delay3/1, Delay2/1, Delay1/1, Delay9/1, Delay8/1, Delay7/1, Delay6/1, MATLAB Function2/1(a), Delay5/1
  Delay8/1 -> MATLAB Function2/5(e)
  Square2/1 -> Relational Operator2/2
  Delay3/1 -> MATLAB Function2/9(ai)
  Delay1/1 -> MATLAB Function2/7(g)
  MATLAB Function2/1(y0) -> Gain1/1
  Delay5/1 -> MATLAB Function2/2(b)
  Product2/1 -> Y2/1
  Delay9/1 -> MATLAB Function2/6(f)
  Delay7/1 -> MATLAB Function2/4(d)
  Constant2/1 -> Relational Operator2/1
  Delay6/1 -> MATLAB Function2/3(c)
  Relational Operator2/1 -> Product2/1, Scope2/1
  Delay4/1 -> MATLAB Function2/10(aj)
  Delay2/1 -> MATLAB Function2/8(h)
  Gain1/1 -> Product2/2, Square2/1

== system fixedWingPath/2ème étage/Test ==
  PosN1 : Inport
  Delay1 : Delay  DelayLength=6  SampleTime=Tgps
  Delay2 : Delay  DelayLength=7  SampleTime=Tgps
  Delay5 : Delay  DelayLength=1  SampleTime=Tgps
  Delay6 : Delay  SampleTime=Tgps
  Delay7 : Delay  DelayLength=3  SampleTime=Tgps
  Delay8 : Delay  DelayLength=4  SampleTime=Tgps
  Delay9 : Delay  DelayLength=5  SampleTime=Tgps
  MATLAB Function2 : MATLAB Function  TreatAsAtomicUnit=on
  y : Outport
  wires:
  PosN1/1 -> Delay2/1, Delay1/1, Delay9/1, Delay8/1, Delay7/1, Delay6/1, Delay5/1, MATLAB Function2/1(a)
  Delay5/1 -> MATLAB Function2/2(b)
  MATLAB Function2/1(y0) -> y/1
  Delay7/1 -> MATLAB Function2/4(d)
  Delay9/1 -> MATLAB Function2/6(f)
  Delay1/1 -> MATLAB Function2/7(g)
  Delay2/1 -> MATLAB Function2/8(h)
  Delay6/1 -> MATLAB Function2/3(c)
  Delay8/1 -> MATLAB Function2/5(e)

== system fixedWingPath/2ème étage/Test1 ==
  PosN1 : Inport
  Delay1 : Delay  DelayLength=6  SampleTime=Tgps
  Delay2 : Delay  DelayLength=7  SampleTime=Tgps
  Delay5 : Delay  DelayLength=1  SampleTime=Tgps
  Delay6 : Delay  SampleTime=Tgps
  Delay7 : Delay  DelayLength=3  SampleTime=Tgps
  Delay8 : Delay  DelayLength=4  SampleTime=Tgps
  Delay9 : Delay  DelayLength=5  SampleTime=Tgps
  MATLAB Function2 : MATLAB Function  TreatAsAtomicUnit=on
  y1 : Outport
  wires:
  PosN1/1 -> Delay2/1, Delay1/1, Delay9/1, Delay8/1, Delay7/1, Delay6/1, Delay5/1, MATLAB Function2/1(a)
  Delay5/1 -> MATLAB Function2/2(b)
  MATLAB Function2/1(y0) -> y1/1
  Delay7/1 -> MATLAB Function2/4(d)
  Delay9/1 -> MATLAB Function2/6(f)
  Delay1/1 -> MATLAB Function2/7(g)
  Delay2/1 -> MATLAB Function2/8(h)
  Delay6/1 -> MATLAB Function2/3(c)
  Delay8/1 -> MATLAB Function2/5(e)

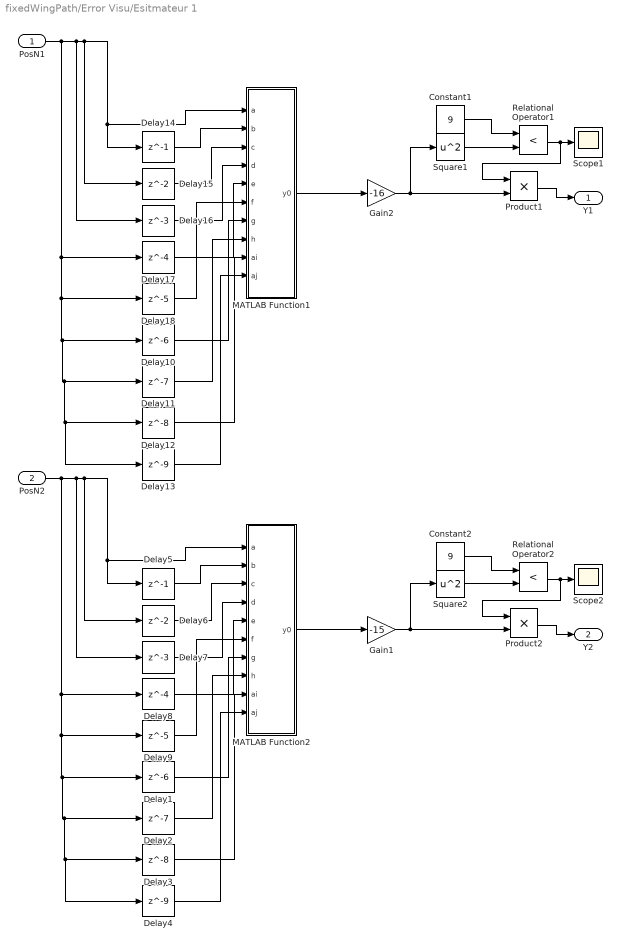
== system fixedWingPath/Error Visu/Esitmateur 1 ==
  PosN1 : Inport
  PosN2 : Inport  Port=2
  Constant1 : Constant  Value=9
  Constant2 : Constant  Value=9
  Delay1 : Delay  DelayLength=6  SampleTime=Tgps
  Delay10 : Delay  DelayLength=6  SampleTime=Tgps
  Delay11 : Delay  DelayLength=7  SampleTime=Tgps
  Delay12 : Delay  DelayLength=8  SampleTime=Tgps
  Delay13 : Delay  DelayLength=9  SampleTime=Tgps
  Delay14 : Delay  DelayLength=1  SampleTime=Tgps
  Delay15 : Delay  SampleTime=Tgps
  Delay16 : Delay  DelayLength=3  SampleTime=Tgps
  Delay17 : Delay  DelayLength=4  SampleTime=Tgps
  Delay18 : Delay  DelayLength=5  SampleTime=Tgps
  Delay2 : Delay  DelayLength=7  SampleTime=Tgps
  Delay3 : Delay  DelayLength=8  SampleTime=Tgps
  Delay4 : Delay  DelayLength=9  SampleTime=Tgps
  Delay5 : Delay  DelayLength=1  SampleTime=Tgps
  Delay6 : Delay  SampleTime=Tgps
  Delay7 : Delay  DelayLength=3  SampleTime=Tgps
  Delay8 : Delay  DelayLength=4  SampleTime=Tgps
  Delay9 : Delay  DelayLength=5  SampleTime=Tgps
  Gain1 : Gain  Gain=-15
  Gain2 : Gain  Gain=-16
  MATLAB Function1 : MATLAB Function  TreatAsAtomicUnit=on
  MATLAB Function2 : MATLAB Function  TreatAsAtomicUnit=on
  Product1 : Product
  Product2 : Product
  Relational Operator1 : RelationalOperator  Operator=<  OutDataTypeStr=boolean  RndMeth=Simplest  InputSameDT=off
  Relational Operator2 : RelationalOperator  Operator=<  OutDataTypeStr=boolean  RndMeth=Simplest  InputSameDT=off
  Scope1 : Scope
  Scope2 : Scope
  Square1 : Math  Operator=square
  Square2 : Math  Operator=square
  Y1 : Outport
  Y2 : Outport  Port=2
  wires:
  Relational Operator1/1 -> Product1/1, Scope1/1
  Constant1/1 -> Relational Operator1/1
  Delay12/1 -> MATLAB Function1/9(ai)
  Delay13/1 -> MATLAB Function1/10(aj)
  Square1/1 -> Relational Operator1/2
  Delay14/1 -> MATLAB Function1/2(b)
  Delay10/1 -> MATLAB Function1/7(g)
  Delay17/1 -> MATLAB Function1/5(e)
  PosN1/1 -> Delay13/1, Delay12/1, Delay11/1, Delay10/1, Delay18/1, Delay17/1, Delay16/1, Delay15/1, MATLAB Function1/1(a), Delay14/1
  Delay11/1 -> MATLAB Function1/8(h)
  Gain2/1 -> Product1/2, Square1/1
  MATLAB Function1/1(y0) -> Gain2/1
  Delay15/1 -> MATLAB Function1/3(c)
  Delay18/1 -> MATLAB Function1/6(f)
  Delay16/1 -> MATLAB Function1/4(d)
  Product1/1 -> Y1/1
  PosN2/1 -> Delay4/1, Delay3/1, Delay2/1, Delay1/1, Delay9/1, Delay8/1, Delay7/1, Delay6/1, MATLAB Function2/1(a), Delay5/1
  Delay8/1 -> MATLAB Function2/5(e)
  Square2/1 -> Relational Operator2/2
  Delay3/1 -> MATLAB Function2/9(ai)
  Delay1/1 -> MATLAB Function2/7(g)
  MATLAB Function2/1(y0) -> Gain1/1
  Delay5/1 -> MATLAB Function2/2(b)
  Product2/1 -> Y2/1
  Delay9/1 -> MATLAB Function2/6(f)
  Delay7/1 -> MATLAB Function2/4(d)
  Constant2/1 -> Relational Operator2/1
  Delay6/1 -> MATLAB Function2/3(c)
  Relational Operator2/1 -> Product2/1, Scope2/1
  Delay4/1 -> MATLAB Function2/10(aj)
  Delay2/1 -> MATLAB Function2/8(h)
  Gain1/1 -> Product2/2, Square2/1

== system fixedWingPath/Esitmateur Traj/Test ==
  PosN1 : Inport
  Delay1 : Delay  DelayLength=6  SampleTime=Tgps
  Delay10 : Delay  DelayLength=10  SampleTime=Tgps
  Delay11 : Delay  DelayLength=11  SampleTime=Tgps
  Delay12 : Delay  DelayLength=12  SampleTime=Tgps
  Delay13 : Delay  DelayLength=13  SampleTime=Tgps
  Delay14 : Delay  DelayLength=14  SampleTime=Tgps
  Delay2 : Delay  DelayLength=7  SampleTime=Tgps
  Delay3 : Delay  DelayLength=8  SampleTime=Tgps
  Delay4 : Delay  DelayLength=9  SampleTime=Tgps
  Delay5 : Delay  DelayLength=1  SampleTime=Tgps
  Delay6 : Delay  SampleTime=Tgps
  Delay7 : Delay  DelayLength=3  SampleTime=Tgps
  Delay8 : Delay  DelayLength=4  SampleTime=Tgps
  Delay9 : Delay  DelayLength=5  SampleTime=Tgps
  MATLAB Function2 : MATLAB Function  TreatAsAtomicUnit=on
  y : Outport
  wires:
  PosN1/1 -> Delay14/1, Delay13/1, Delay12/1, Delay11/1, Delay10/1, Delay4/1, Delay3/1, Delay2/1, Delay1/1, Delay9/1, Delay8/1, Delay7/1, Delay6/1, Delay5/1, MATLAB Function2/1(a)
  Delay5/1 -> MATLAB Function2/2(b)
  MATLAB Function2/1(y0) -> y/1
  Delay7/1 -> MATLAB Function2/4(d)
  Delay9/1 -> MATLAB Function2/6(f)
  Delay1/1 -> MATLAB Function2/7(g)
  Delay2/1 -> MATLAB Function2/8(h)
  Delay6/1 -> MATLAB Function2/3(c)
  Delay8/1 -> MATLAB Function2/5(e)
  Delay3/1 -> MATLAB Function2/9(ii)
  Delay4/1 -> MATLAB Function2/10(jj)
  Delay10/1 -> MATLAB Function2/11(k)
  Delay11/1 -> MATLAB Function2/12(l)
  Delay12/1 -> MATLAB Function2/13(m)
  Delay13/1 -> MATLAB Function2/14(n)
  Delay14/1 -> MATLAB Function2/15(o)

== system fixedWingPath/Esitmateur Traj/Test1 ==
  PosN1 : Inport
  Delay1 : Delay  DelayLength=6  SampleTime=Tgps
  Delay10 : Delay  DelayLength=10  SampleTime=Tgps
  Delay11 : Delay  DelayLength=11  SampleTime=Tgps
  Delay12 : Delay  DelayLength=12  SampleTime=Tgps
  Delay13 : Delay  DelayLength=13  SampleTime=Tgps
  Delay14 : Delay  DelayLength=14  SampleTime=Tgps
  Delay2 : Delay  DelayLength=7  SampleTime=Tgps
  Delay3 : Delay  DelayLength=8  SampleTime=Tgps
  Delay4 : Delay  DelayLength=9  SampleTime=Tgps
  Delay5 : Delay  DelayLength=1  SampleTime=Tgps
  Delay6 : Delay  SampleTime=Tgps
  Delay7 : Delay  DelayLength=3  SampleTime=Tgps
  Delay8 : Delay  DelayLength=4  SampleTime=Tgps
  Delay9 : Delay  DelayLength=5  SampleTime=Tgps
  MATLAB Function2 : MATLAB Function  TreatAsAtomicUnit=on
  y : Outport
  wires:
  PosN1/1 -> Delay14/1, Delay13/1, Delay12/1, Delay11/1, Delay10/1, Delay4/1, Delay3/1, Delay2/1, Delay1/1, Delay9/1, Delay8/1, Delay7/1, Delay6/1, Delay5/1, MATLAB Function2/1(a)
  Delay5/1 -> MATLAB Function2/2(b)
  MATLAB Function2/1(y0) -> y/1
  Delay7/1 -> MATLAB Function2/4(d)
  Delay9/1 -> MATLAB Function2/6(f)
  Delay1/1 -> MATLAB Function2/7(g)
  Delay2/1 -> MATLAB Function2/8(h)
  Delay6/1 -> MATLAB Function2/3(c)
  Delay8/1 -> MATLAB Function2/5(e)
  Delay3/1 -> MATLAB Function2/9(ii)
  Delay4/1 -> MATLAB Function2/10(jj)
  Delay10/1 -> MATLAB Function2/11(k)
  Delay11/1 -> MATLAB Function2/12(l)
  Delay12/1 -> MATLAB Function2/13(m)
  Delay13/1 -> MATLAB Function2/14(n)
  Delay14/1 -> MATLAB Function2/15(o)

== system fixedWingPath/Esitmateur Traj1/Test ==
  PosN1 : Inport
  Delay1 : Delay  DelayLength=6  SampleTime=Tgps
  Delay10 : Delay  DelayLength=10  SampleTime=Tgps
  Delay11 : Delay  DelayLength=11  SampleTime=Tgps
  Delay12 : Delay  DelayLength=12  SampleTime=Tgps
  Delay13 : Delay  DelayLength=13  SampleTime=Tgps
  Delay14 : Delay  DelayLength=14  SampleTime=Tgps
  Delay2 : Delay  DelayLength=7  SampleTime=Tgps
  Delay3 : Delay  DelayLength=8  SampleTime=Tgps
  Delay4 : Delay  DelayLength=9  SampleTime=Tgps
  Delay5 : Delay  DelayLength=1  SampleTime=Tgps
  Delay6 : Delay  SampleTime=Tgps
  Delay7 : Delay  DelayLength=3  SampleTime=Tgps
  Delay8 : Delay  DelayLength=4  SampleTime=Tgps
  Delay9 : Delay  DelayLength=5  SampleTime=Tgps
  MATLAB Function2 : MATLAB Function  TreatAsAtomicUnit=on
  y : Outport
  wires:
  PosN1/1 -> Delay14/1, Delay13/1, Delay12/1, Delay11/1, Delay10/1, Delay4/1, Delay3/1, Delay2/1, Delay1/1, Delay9/1, Delay8/1, Delay7/1, Delay6/1, Delay5/1, MATLAB Function2/1(a)
  Delay5/1 -> MATLAB Function2/2(b)
  MATLAB Function2/1(y0) -> y/1
  Delay7/1 -> MATLAB Function2/4(d)
  Delay9/1 -> MATLAB Function2/6(f)
  Delay1/1 -> MATLAB Function2/7(g)
  Delay2/1 -> MATLAB Function2/8(h)
  Delay6/1 -> MATLAB Function2/3(c)
  Delay8/1 -> MATLAB Function2/5(e)
  Delay3/1 -> MATLAB Function2/9(ii)
  Delay4/1 -> MATLAB Function2/10(jj)
  Delay10/1 -> MATLAB Function2/11(k)
  Delay11/1 -> MATLAB Function2/12(l)
  Delay12/1 -> MATLAB Function2/13(m)
  Delay13/1 -> MATLAB Function2/14(n)
  Delay14/1 -> MATLAB Function2/15(o)

== system fixedWingPath/Esitmateur Traj1/Test2 ==
  PosN1 : Inport
  Delay1 : Delay  DelayLength=6  SampleTime=Tgps
  Delay10 : Delay  DelayLength=10  SampleTime=Tgps
  Delay11 : Delay  DelayLength=11  SampleTime=Tgps
  Delay12 : Delay  DelayLength=12  SampleTime=Tgps
  Delay13 : Delay  DelayLength=13  SampleTime=Tgps
  Delay14 : Delay  DelayLength=14  SampleTime=Tgps
  Delay2 : Delay  DelayLength=7  SampleTime=Tgps
  Delay3 : Delay  DelayLength=8  SampleTime=Tgps
  Delay4 : Delay  DelayLength=9  SampleTime=Tgps
  Delay5 : Delay  DelayLength=1  SampleTime=Tgps
  Delay6 : Delay  SampleTime=Tgps
  Delay7 : Delay  DelayLength=3  SampleTime=Tgps
  Delay8 : Delay  DelayLength=4  SampleTime=Tgps
  Delay9 : Delay  DelayLength=5  SampleTime=Tgps
  MATLAB Function2 : MATLAB Function  TreatAsAtomicUnit=on
  y : Outport
  wires:
  PosN1/1 -> Delay14/1, Delay13/1, Delay12/1, Delay11/1, Delay10/1, Delay4/1, Delay3/1, Delay2/1, Delay1/1, Delay9/1, Delay8/1, Delay7/1, Delay6/1, Delay5/1, MATLAB Function2/1(a)
  Delay5/1 -> MATLAB Function2/2(b)
  MATLAB Function2/1(y0) -> y/1
  Delay7/1 -> MATLAB Function2/4(d)
  Delay9/1 -> MATLAB Function2/6(f)
  Delay1/1 -> MATLAB Function2/7(g)
  Delay2/1 -> MATLAB Function2/8(h)
  Delay6/1 -> MATLAB Function2/3(c)
  Delay8/1 -> MATLAB Function2/5(e)
  Delay3/1 -> MATLAB Function2/9(ii)
  Delay4/1 -> MATLAB Function2/10(jj)
  Delay10/1 -> MATLAB Function2/11(k)
  Delay11/1 -> MATLAB Function2/12(l)
  Delay12/1 -> MATLAB Function2/13(m)
  Delay13/1 -> MATLAB Function2/14(n)
  Delay14/1 -> MATLAB Function2/15(o)

== system fixedWingPath/Windless/WIND GENERATOR ==
  Gain : Gain  Gain=5
  Random Number : RandomNumber  Variance=1*VarNeuro  SampleTime=0.1
  Transfer Fcn : TransferFcn  Numerator=[10000]  Denominator=[10000 0.01]
  Out1 : Outport
  wires:
  Gain/1 -> Out1/1
  Transfer Fcn/1 -> Gain/1
  Random Number/1 -> Transfer Fcn/1

== system fixedWingPath/Windless/WIND GENERATOR1 ==
  Gain : Gain  Gain=5
  Random Number : RandomNumber  Variance=1*VarNeuro  SampleTime=0.1
  Transfer Fcn : TransferFcn  Numerator=[10000]  Denominator=[10000 0.01]
  Out1 : Outport
  wires:
  Gain/1 -> Out1/1
  Transfer Fcn/1 -> Gain/1
  Random Number/1 -> Transfer Fcn/1

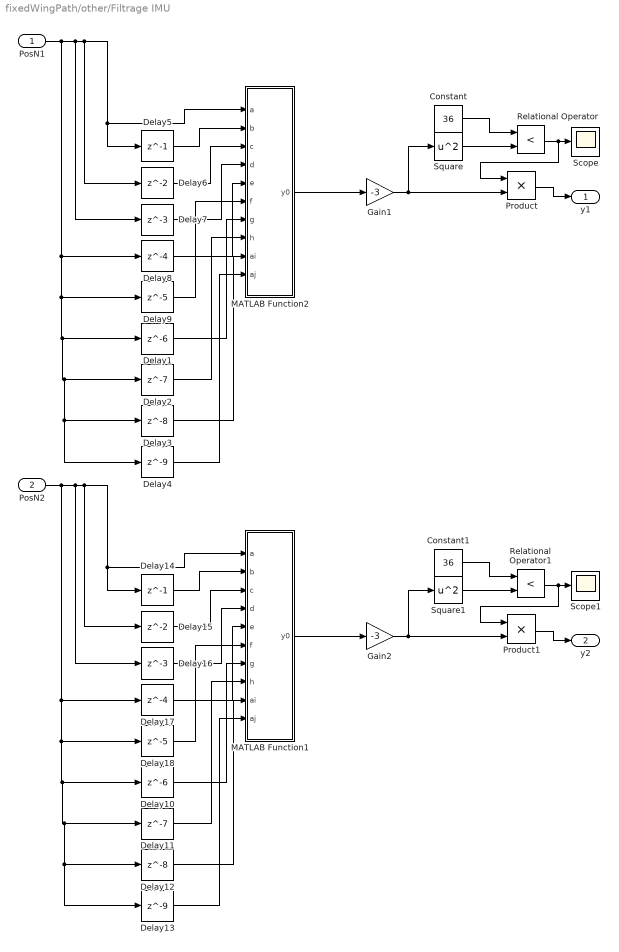
== system fixedWingPath/other/Filtrage IMU ==
  PosN1 : Inport
  PosN2 : Inport  Port=2
  Constant : Constant  Value=36
  Constant1 : Constant  Value=36
  Delay1 : Delay  DelayLength=6  SampleTime=Tgps
  Delay10 : Delay  DelayLength=6  SampleTime=Tgps
  Delay11 : Delay  DelayLength=7  SampleTime=Tgps
  Delay12 : Delay  DelayLength=8  SampleTime=Tgps
  Delay13 : Delay  DelayLength=9  SampleTime=Tgps
  Delay14 : Delay  DelayLength=1  SampleTime=Tgps
  Delay15 : Delay  SampleTime=Tgps
  Delay16 : Delay  DelayLength=3  SampleTime=Tgps
  Delay17 : Delay  DelayLength=4  SampleTime=Tgps
  Delay18 : Delay  DelayLength=5  SampleTime=Tgps
  Delay2 : Delay  DelayLength=7  SampleTime=Tgps
  Delay3 : Delay  DelayLength=8  SampleTime=Tgps
  Delay4 : Delay  DelayLength=9  SampleTime=Tgps
  Delay5 : Delay  DelayLength=1  SampleTime=Tgps
  Delay6 : Delay  SampleTime=Tgps
  Delay7 : Delay  DelayLength=3  SampleTime=Tgps
  Delay8 : Delay  DelayLength=4  SampleTime=Tgps
  Delay9 : Delay  DelayLength=5  SampleTime=Tgps
  Gain1 : Gain  Gain=-3
  Gain2 : Gain  Gain=-3
  MATLAB Function1 : MATLAB Function  TreatAsAtomicUnit=on
  MATLAB Function2 : MATLAB Function  TreatAsAtomicUnit=on
  Product : Product
  Product1 : Product
  Relational Operator : RelationalOperator  Operator=<  OutDataTypeStr=boolean  RndMeth=Simplest  InputSameDT=off
  Relational Operator1 : RelationalOperator  Operator=<  OutDataTypeStr=boolean  RndMeth=Simplest  InputSameDT=off
  Scope : Scope
  Scope1 : Scope
  Square : Math  Operator=square
  Square1 : Math  Operator=square
  y1 : Outport
  y2 : Outport  Port=2
  wires:
  PosN1/1 -> Delay4/1, Delay3/1, Delay2/1, Delay1/1, Delay9/1, Delay8/1, Delay7/1, Delay6/1, MATLAB Function2/1(a), Delay5/1
  Delay5/1 -> MATLAB Function2/2(b)
  Delay6/1 -> MATLAB Function2/3(c)
  Delay7/1 -> MATLAB Function2/4(d)
  Delay8/1 -> MATLAB Function2/5(e)
  Delay9/1 -> MATLAB Function2/6(f)
  Gain1/1 -> Product/2, Square/1
  MATLAB Function2/1(y0) -> Gain1/1
  Delay1/1 -> MATLAB Function2/7(g)
  Delay2/1 -> MATLAB Function2/8(h)
  Delay3/1 -> MATLAB Function2/9(ai)
  Delay4/1 -> MATLAB Function2/10(aj)
  Constant/1 -> Relational Operator/1
  Square/1 -> Relational Operator/2
  Relational Operator/1 -> Product/1, Scope/1
  Product/1 -> y1/1
  Relational Operator1/1 -> Product1/1, Scope1/1
  Constant1/1 -> Relational Operator1/1
  Delay12/1 -> MATLAB Function1/9(ai)
  Delay13/1 -> MATLAB Function1/10(aj)
  Square1/1 -> Relational Operator1/2
  Delay14/1 -> MATLAB Function1/2(b)
  Delay10/1 -> MATLAB Function1/7(g)
  Delay17/1 -> MATLAB Function1/5(e)
  PosN2/1 -> Delay13/1, Delay12/1, Delay11/1, Delay10/1, Delay18/1, Delay17/1, Delay16/1, Delay15/1, MATLAB Function1/1(a), Delay14/1
  Delay11/1 -> MATLAB Function1/8(h)
  Gain2/1 -> Product1/2, Square1/1
  MATLAB Function1/1(y0) -> Gain2/1
  Delay15/1 -> MATLAB Function1/3(c)
  Delay18/1 -> MATLAB Function1/6(f)
  Delay16/1 -> MATLAB Function1/4(d)
  Product1/1 -> y2/1

== matlab function fixedWingPath/other/Filtrage IMU/MATLAB Function1 ==
  data: a input; y0 output; b input; c input; d input; e input; f input; g input; h input; ai input; aj input
function y0   = fcn(a, b, c, d, e, f, g ,h , ai, aj)
%temps =[0 1 2 3 4 5];
%elevation =[f e d c b a];
temps =[0 1 2 3 4 5 6 7 8];
elevation =[aj ai h g f e d c b a];

Delay = 0;

windowSize = 9;
elevation_smoothed = movmean(elevation, windowSize);


y0 = elevation_smoothed(5);

== matlab function fixedWingPath/other/Filtrage IMU/MATLAB Function2 ==
  data: a input; y0 output; b input; c input; d input; e input; f input; g input; h input; ai input; aj input
function y0   = fcn(a, b, c, d, e, f, g ,h , ai, aj)
%temps =[0 1 2 3 4 5];
%elevation =[f e d c b a];
temps =[0 1 2 3 4 5 6 7 8];
elevation =[aj ai h g f e d c b a];

Delay = 0;

windowSize = 9;
elevation_smoothed = movmean(elevation, windowSize);


y0 = elevation_smoothed(5);

== matlab function fixedWingPath/2ème étage/Test/MATLAB Function2 ==
  data: a input; y0 output; b input; c input; d input; e input; f input; g input; h input
function y0   = fcn(a, b, c, d, e, f, g ,h)
%temps =[0 1 2 3 4 5];
%elevation =[f e d c b a];
temps =[0 1 2 3 4 5 6 7];
elevation =[h g f e d c b a];

Delay = 0;

windowSize = 5;
elevation_smoothed = movmean(elevation, windowSize);


y0 = elevation_smoothed(8);

== matlab function fixedWingPath/2ème étage/Test1/MATLAB Function2 ==
  data: a input; y0 output; b input; c input; d input; e input; f input; g input; h input
function y0   = fcn(a, b, c, d, e, f, g ,h)
%temps =[0 1 2 3 4 5];
%elevation =[f e d c b a];
temps =[0 1 2 3 4 5 6 7];
elevation =[h g f e d c b a];

Delay = 0;

windowSize = 5;
elevation_smoothed = movmean(elevation, windowSize);


y0 = elevation_smoothed(8);

== matlab function fixedWingPath/Error Visu/Esitmateur 1/MATLAB Function1 ==
  data: a input; y0 output; b input; c input; d input; e input; f input; g input; h input; ai input; aj input
function y0   = fcn(a, b, c, d, e, f, g ,h , ai, aj)
%temps =[0 1 2 3 4 5];
%elevation =[f e d c b a];
temps =[0 1 2 3 4 5 6 7 8];
elevation =[aj ai h g f e d c b a];

Delay = 0;

windowSize = 9;
elevation_smoothed = movmean(elevation, windowSize);


y0 = elevation_smoothed(7);

== matlab function fixedWingPath/2ème étage/Esitmateur 1/MATLAB Function2 ==
  data: a input; y0 output; b input; c input; d input; e input; f input; g input; h input; ai input; aj input
function y0   = fcn(a, b, c, d, e, f, g ,h , ai, aj)
%temps =[0 1 2 3 4 5];
%elevation =[f e d c b a];
temps =[0 1 2 3 4 5 6 7 8 9];
elevation =[aj ai h g f e d c b a];

Delay = 0;

windowSize = 9;
elevation_smoothed = movmean(elevation, windowSize);


y0 = elevation_smoothed(9);

== matlab function fixedWingPath/Esitmateur Traj/Test1/MATLAB Function2 ==
  data: a input; y0 output; b input; c input; d input; e input; f input; g input; h input; ii input; jj input; k input; l input; m input; n input; o input
function y0   = fcn(a, b, c, d, e, f, g ,h, ii, jj, k, l, m, n, o)
%temps =[0 1 2 3 4 5];
%elevation =[f e d c b a];
temps =[0 1 2 3 4 5 6 7 8 9 10 11 12 13 14];
elevation =[o n m l k jj ii h g f e d c b a];

windowSize = 15; %filtrage sur 3s
%elevation_sg = sgolayfilt(elevation, 2 ,windowSize);
elevation_smoothed = movmean(elevation, windowSize);

%weights = linspace(1, 0, windowSize);


y0 = elevation_smoothed(15);
